simulink model "SYSTEMCOMPLEX"  (R2025b)
settings: Solver=VariableStepAuto  StartTime=0.0  StopTime=10.0  RelTol=1e-3
(part 1 of 2)
settings Model: Creator=GShelton28  LastModifiedBy=GShelton28

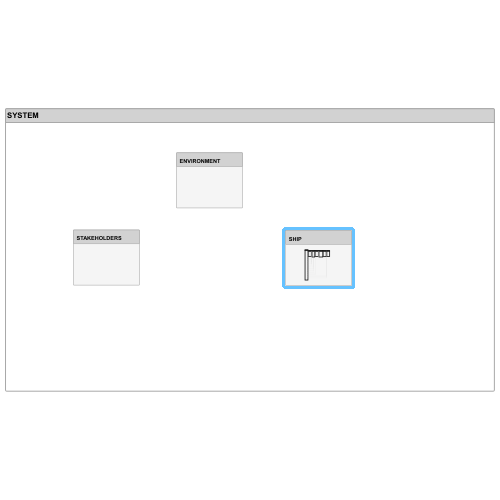
[thumbnail: Simulink's stored preview of the top-level diagram]
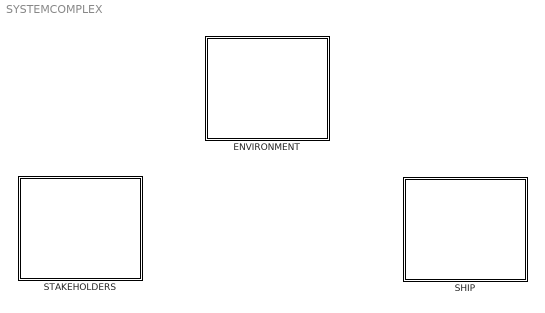
== system SYSTEMCOMPLEX ==
  ENVIRONMENT : Subsystem
      settings: PortSchema="{\"entries\":[{\"content\":{\"headerSize\":26,\"margin\":15,\"minimumSpacing\":25,\"sides\":[{\"content\":{},\"type\":\"ConnectorPlacement.EquallySpacedRectSide\",\"uuid\":\"c62bca68-e99b-4d4a-8c3b-c9a3c6520291\"},{\"content\":{\"side\":\"RIGHT\"},\"type\":\"ConnectorPlacement.EquallySpacedRectSide\",\"uuid\":\"9f78cd75-5645-4950-8d66-9f0d33627f1f\"},{\"content\":{\"side\":\"TOP\"},\"type\":\"ConnectorPlacement.EquallySpacedRectSide\",\"uuid\":\"f95077c9-4a6b-4bf1-8b13-59697d659817\"}]},\"type\":\"ConnectorPlacement.EquallySpacedConnector\",\"uuid\":\"da1ef182-4ed3-4fb4-823f-e8eb0a5ecd15\"}],\"packageUris\":[\"http://schema.mathworks.com/mf0/Connector/R2020b\"],\"version\":\"1.0\"}"
  SHIP : Subsystem
      settings: PortSchema="{\"entries\":[{\"content\":{\"headerSize\":26,\"margin\":15,\"minimumSpacing\":25,\"sides\":[{\"content\":{},\"type\":\"ConnectorPlacement.EquallySpacedRectSide\",\"uuid\":\"c62bca68-e99b-4d4a-8c3b-c9a3c6520291\"},{\"content\":{\"side\":\"RIGHT\"},\"type\":\"ConnectorPlacement.EquallySpacedRectSide\",\"uuid\":\"9f78cd75-5645-4950-8d66-9f0d33627f1f\"},{\"content\":{\"side\":\"TOP\"},\"type\":\"ConnectorPlacement.EquallySpacedRectSide\",\"uuid\":\"f95077c9-4a6b-4bf1-8b13-59697d659817\"}]},\"type\":\"ConnectorPlacement.EquallySpacedConnector\",\"uuid\":\"da1ef182-4ed3-4fb4-823f-e8eb0a5ecd15\"}],\"packageUris\":[\"http://schema.mathworks.com/mf0/Connector/R2020b\"],\"version\":\"1.0\"}"
  STAKEHOLDERS : Subsystem
      settings: PortSchema="{\"entries\":[{\"content\":{\"headerSize\":26,\"margin\":15,\"minimumSpacing\":25,\"sides\":[{\"content\":{},\"type\":\"ConnectorPlacement.EquallySpacedRectSide\",\"uuid\":\"c62bca68-e99b-4d4a-8c3b-c9a3c6520291\"},{\"content\":{\"side\":\"RIGHT\"},\"type\":\"ConnectorPlacement.EquallySpacedRectSide\",\"uuid\":\"9f78cd75-5645-4950-8d66-9f0d33627f1f\"},{\"content\":{\"side\":\"TOP\"},\"type\":\"ConnectorPlacement.EquallySpacedRectSide\",\"uuid\":\"f95077c9-4a6b-4bf1-8b13-59697d659817\"}]},\"type\":\"ConnectorPlacement.EquallySpacedConnector\",\"uuid\":\"da1ef182-4ed3-4fb4-823f-e8eb0a5ecd15\"}],\"packageUris\":[\"http://schema.mathworks.com/mf0/Connector/R2020b\"],\"version\":\"1.0\"}"

== system SYSTEMCOMPLEX/ENVIRONMENT ==

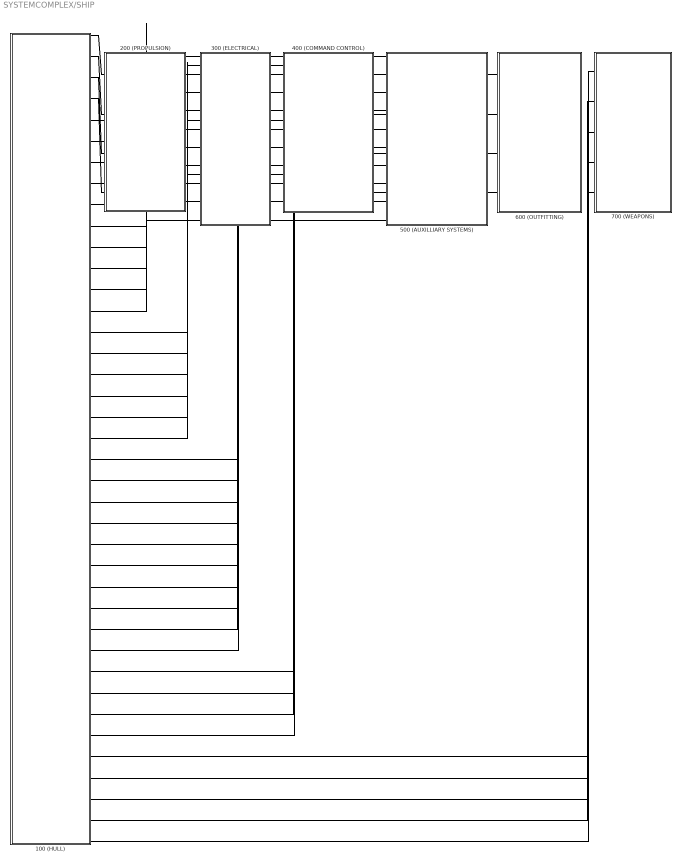
== system SYSTEMCOMPLEX/SHIP ==
  100 (HULL) : Subsystem
      settings: PortSchema="{\"entries\":[{\"content\":{\"headerSize\":26,\"margin\":15,\"minimumSpacing\":25,\"sides\":[{\"content\":{},\"type\":\"ConnectorPlacement.EquallySpacedRectSide\",\"uuid\":\"c62bca68-e99b-4d4a-8c3b-c9a3c6520291\"},{\"content\":{\"connectorIds\":[\"RConn1\",\"RConn2\",\"RConn3\",\"RConn4\",\"RConn5\",\"RConn6\",\"RConn7\",\"RConn8\",\"RConn9\",\"RConn10\",\"RConn11\",\"RConn12\",\"RConn13\",\"RConn14\",\"RConn15\",\"RConn16\",\"RConn17\",\"RConn18\",\"RConn19\",\"RConn20\",\"RConn21\",\"RConn22\",\"RConn23\",\"RConn24\",\"RConn25\",\"RConn26\",\"RConn27\",\"RConn28\",\"RConn29\",\"RConn30\",\"RConn31\",\"RConn32\",\"RConn33\",\"RConn34\",\"RConn35\",\"RConn36\",\"RConn37\",\"RConn38\",\"RConn39\"],\"side\":\"RIGHT\"},\"type\":\"ConnectorPlacement.EquallySpacedRectSide\",\"uuid\":\"9f78cd75-5645-4950-8d66-9f0d33627f1f\"},{\"content\":{\"side\":\"TOP\"},\"type\":\"ConnectorPlacement.EquallySpacedRectSide\",\"uuid\":\"f95077c9-4a6b-4bf1-8b13-59697d659817\"}]},\"type\":\"ConnectorPlacement.EquallySpacedConnector\",\"uuid\":\"da1ef182-4ed3-4fb4-823f-e8eb0a5ecd15\"}],\"packageUris\":[\"http://schema.mathworks.com/mf0/Connector/R2020b\"],\"version\":\"1.0\"}"
  200 (PROPULSION) : Subsystem
      settings: PortSchema="{\"entries\":[{\"content\":{\"headerSize\":26,\"margin\":15,\"minimumSpacing\":25,\"sides\":[{\"content\":{\"connectorIds\":[\"LConn1\",\"LConn2\",\"LConn3\",\"LConn4\"]},\"type\":\"ConnectorPlacement.EquallySpacedRectSide\",\"uuid\":\"c62bca68-e99b-4d4a-8c3b-c9a3c6520291\"},{\"content\":{\"side\":\"RIGHT\"},\"type\":\"ConnectorPlacement.EquallySpacedRectSide\",\"uuid\":\"9f78cd75-5645-4950-8d66-9f0d33627f1f\"},{\"content\":{\"side\":\"TOP\"},\"type\":\"ConnectorPlacement.EquallySpacedRectSide\",\"uuid\":\"f95077c9-4a6b-4bf1-8b13-59697d659817\"}]},\"type\":\"ConnectorPlacement.EquallySpacedConnector\",\"uuid\":\"da1ef182-4ed3-4fb4-823f-e8eb0a5ecd15\"}],\"packageUris\":[\"http://schema.mathworks.com/mf0/Connector/R2020b\"],\"version\":\"1.0\"}"
  300 (ELECTRICAL) : Subsystem
      settings: PortSchema="{\"entries\":[{\"content\":{\"headerSize\":26,\"margin\":15,\"minimumSpacing\":25,\"sides\":[{\"content\":{\"connectorIds\":[\"LConn1\",\"LConn2\",\"LConn3\",\"LConn4\",\"LConn5\",\"LConn6\",\"LConn7\",\"LConn8\",\"LConn9\",\"LConn10\"]},\"type\":\"ConnectorPlacement.EquallySpacedRectSide\",\"uuid\":\"c62bca68-e99b-4d4a-8c3b-c9a3c6520291\"},{\"content\":{\"side\":\"RIGHT\"},\"type\":\"ConnectorPlacement.EquallySpacedRectSide\",\"uuid\":\"9f78cd75-5645-4950-8d66-9f0d33627f1f\"},{\"content\":{\"side\":\"TOP\"},\"type\":\"ConnectorPlacement.EquallySpacedRectSide\",\"uuid\":\"f95077c9-4a6b-4bf1-8b13-59697d659817\"}]},\"type\":\"ConnectorPlacement.EquallySpacedConnector\",\"uuid\":\"da1ef182-4ed3-4fb4-823f-e8eb0a5ecd15\"}],\"packageUris\":[\"http://schema.mathworks.com/mf0/Connector/R2020b\"],\"version\":\"1.0\"}"
  400 (COMMAND CONTROL) : Subsystem
      settings: PortSchema="{\"entries\":[{\"content\":{\"headerSize\":26,\"margin\":15,\"minimumSpacing\":25,\"sides\":[{\"content\":{\"connectorIds\":[\"LConn1\",\"LConn2\",\"LConn3\",\"LConn4\",\"LConn5\",\"LConn6\"]},\"type\":\"ConnectorPlacement.EquallySpacedRectSide\",\"uuid\":\"c62bca68-e99b-4d4a-8c3b-c9a3c6520291\"},{\"content\":{\"side\":\"RIGHT\"},\"type\":\"ConnectorPlacement.EquallySpacedRectSide\",\"uuid\":\"9f78cd75-5645-4950-8d66-9f0d33627f1f\"},{\"content\":{\"side\":\"TOP\"},\"type\":\"ConnectorPlacement.EquallySpacedRectSide\",\"uuid\":\"f95077c9-4a6b-4bf1-8b13-59697d659817\"}]},\"type\":\"ConnectorPlacement.EquallySpacedConnector\",\"uuid\":\"da1ef182-4ed3-4fb4-823f-e8eb0a5ecd15\"}],\"packageUris\":[\"http://schema.mathworks.com/mf0/Connector/R2020b\"],\"version\":\"1.0\"}"
  500 (AUXILLIARY SYSTEMS) : Subsystem
      settings: PortSchema="{\"entries\":[{\"content\":{\"headerSize\":26,\"margin\":15,\"minimumSpacing\":25,\"sides\":[{\"content\":{\"connectorIds\":[\"LConn1\",\"LConn2\",\"LConn3\",\"LConn4\",\"LConn5\",\"LConn6\",\"LConn7\",\"LConn8\",\"LConn9\",\"LConn10\"]},\"type\":\"ConnectorPlacement.EquallySpacedRectSide\",\"uuid\":\"c62bca68-e99b-4d4a-8c3b-c9a3c6520291\"},{\"content\":{\"side\":\"RIGHT\"},\"type\":\"ConnectorPlacement.EquallySpacedRectSide\",\"uuid\":\"9f78cd75-5645-4950-8d66-9f0d33627f1f\"},{\"content\":{\"side\":\"TOP\"},\"type\":\"ConnectorPlacement.EquallySpacedRectSide\",\"uuid\":\"f95077c9-4a6b-4bf1-8b13-59697d659817\"}]},\"type\":\"ConnectorPlacement.EquallySpacedConnector\",\"uuid\":\"da1ef182-4ed3-4fb4-823f-e8eb0a5ecd15\"}],\"packageUris\":[\"http://schema.mathworks.com/mf0/Connector/R2020b\"],\"version\":\"1.0\"}"
  600 (OUTFITTING) : Subsystem
      settings: PortSchema="{\"entries\":[{\"content\":{\"headerSize\":26,\"margin\":15,\"minimumSpacing\":25,\"sides\":[{\"content\":{\"connectorIds\":[\"LConn1\",\"LConn2\",\"LConn3\",\"LConn4\"]},\"type\":\"ConnectorPlacement.EquallySpacedRectSide\",\"uuid\":\"c62bca68-e99b-4d4a-8c3b-c9a3c6520291\"},{\"content\":{\"side\":\"RIGHT\"},\"type\":\"ConnectorPlacement.EquallySpacedRectSide\",\"uuid\":\"9f78cd75-5645-4950-8d66-9f0d33627f1f\"},{\"content\":{\"side\":\"TOP\"},\"type\":\"ConnectorPlacement.EquallySpacedRectSide\",\"uuid\":\"f95077c9-4a6b-4bf1-8b13-59697d659817\"}]},\"type\":\"ConnectorPlacement.EquallySpacedConnector\",\"uuid\":\"da1ef182-4ed3-4fb4-823f-e8eb0a5ecd15\"}],\"packageUris\":[\"http://schema.mathworks.com/mf0/Connector/R2020b\"],\"version\":\"1.0\"}"
  700 (WEAPONS) : Subsystem
      settings: PortSchema="{\"entries\":[{\"content\":{\"headerSize\":26,\"margin\":15,\"minimumSpacing\":25,\"sides\":[{\"content\":{\"connectorIds\":[\"LConn1\",\"LConn2\",\"LConn3\",\"LConn4\",\"LConn5\"]},\"type\":\"ConnectorPlacement.EquallySpacedRectSide\",\"uuid\":\"c62bca68-e99b-4d4a-8c3b-c9a3c6520291\"},{\"content\":{\"side\":\"RIGHT\"},\"type\":\"ConnectorPlacement.EquallySpacedRectSide\",\"uuid\":\"9f78cd75-5645-4950-8d66-9f0d33627f1f\"},{\"content\":{\"side\":\"TOP\"},\"type\":\"ConnectorPlacement.EquallySpacedRectSide\",\"uuid\":\"f95077c9-4a6b-4bf1-8b13-59697d659817\"}]},\"type\":\"ConnectorPlacement.EquallySpacedConnector\",\"uuid\":\"da1ef182-4ed3-4fb4-823f-e8eb0a5ecd15\"}],\"packageUris\":[\"http://schema.mathworks.com/mf0/Connector/R2020b\"],\"version\":\"1.0\"}"
  connections:
  100 (HULL)/RConn1 -- 200 (PROPULSION)/LConn1
  100 (HULL)/RConn2 -- 200 (PROPULSION)/LConn2
  100 (HULL)/RConn3 -- 200 (PROPULSION)/LConn3
  100 (HULL)/RConn4 -- 200 (PROPULSION)/LConn4
  100 (HULL)/RConn5 -- 300 (ELECTRICAL)/LConn1
  100 (HULL)/RConn6 -- 300 (ELECTRICAL)/LConn2
  100 (HULL)/RConn7 -- 300 (ELECTRICAL)/LConn3
  100 (HULL)/RConn8 -- 300 (ELECTRICAL)/LConn4
  100 (HULL)/RConn9 -- 300 (ELECTRICAL)/LConn5
  100 (HULL)/RConn10 -- 300 (ELECTRICAL)/LConn6
  100 (HULL)/RConn11 -- 300 (ELECTRICAL)/LConn7
  100 (HULL)/RConn12 -- 300 (ELECTRICAL)/LConn8
  100 (HULL)/RConn13 -- 300 (ELECTRICAL)/LConn9
  100 (HULL)/RConn14 -- 300 (ELECTRICAL)/LConn10
  100 (HULL)/RConn15 -- 400 (COMMAND CONTROL)/LConn1
  100 (HULL)/RConn16 -- 400 (COMMAND CONTROL)/LConn2
  100 (HULL)/RConn17 -- 400 (COMMAND CONTROL)/LConn3
  100 (HULL)/RConn18 -- 400 (COMMAND CONTROL)/LConn4
  100 (HULL)/RConn19 -- 400 (COMMAND CONTROL)/LConn5
  100 (HULL)/RConn20 -- 400 (COMMAND CONTROL)/LConn6
  500 (AUXILLIARY SYSTEMS)/LConn1 -- 100 (HULL)/RConn21
  100 (HULL)/RConn22 -- 500 (AUXILLIARY SYSTEMS)/LConn2
  100 (HULL)/RConn23 -- 500 (AUXILLIARY SYSTEMS)/LConn3
  100 (HULL)/RConn24 -- 500 (AUXILLIARY SYSTEMS)/LConn4
  500 (AUXILLIARY SYSTEMS)/LConn5 -- 100 (HULL)/RConn25
  100 (HULL)/RConn26 -- 500 (AUXILLIARY SYSTEMS)/LConn6
  500 (AUXILLIARY SYSTEMS)/LConn7 -- 100 (HULL)/RConn27
  100 (HULL)/RConn28 -- 500 (AUXILLIARY SYSTEMS)/LConn8
  500 (AUXILLIARY SYSTEMS)/LConn9 -- 100 (HULL)/RConn29
  100 (HULL)/RConn30 -- 500 (AUXILLIARY SYSTEMS)/LConn10
  600 (OUTFITTING)/LConn1 -- 100 (HULL)/RConn31
  100 (HULL)/RConn32 -- 600 (OUTFITTING)/LConn2
  600 (OUTFITTING)/LConn3 -- 100 (HULL)/RConn33
  100 (HULL)/RConn34 -- 600 (OUTFITTING)/LConn4
  100 (HULL)/RConn35 -- 700 (WEAPONS)/LConn1
  700 (WEAPONS)/LConn2 -- 100 (HULL)/RConn36
  100 (HULL)/RConn37 -- 700 (WEAPONS)/LConn3
  700 (WEAPONS)/LConn4 -- 100 (HULL)/RConn38
  100 (HULL)/RConn39 -- 700 (WEAPONS)/LConn5

== system SYSTEMCOMPLEX/STAKEHOLDERS ==

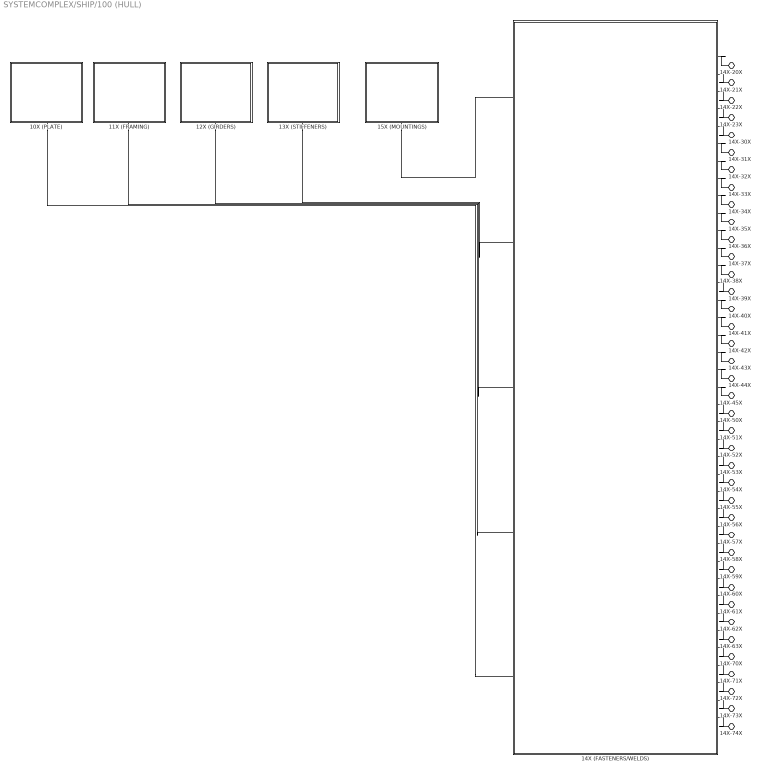
== system SYSTEMCOMPLEX/SHIP/100 (HULL) ==
  10X (PLATE) : Subsystem
      settings: PortSchema="{\"entries\":[{\"content\":{\"headerSize\":26,\"margin\":15,\"minimumSpacing\":25,\"sides\":[{\"content\":{},\"type\":\"ConnectorPlacement.EquallySpacedRectSide\",\"uuid\":\"c62bca68-e99b-4d4a-8c3b-c9a3c6520291\"},{\"content\":{\"side\":\"RIGHT\"},\"type\":\"ConnectorPlacement.EquallySpacedRectSide\",\"uuid\":\"9f78cd75-5645-4950-8d66-9f0d33627f1f\"},{\"content\":{\"side\":\"TOP\"},\"type\":\"ConnectorPlacement.EquallySpacedRectSide\",\"uuid\":\"f95077c9-4a6b-4bf1-8b13-59697d659817\"},{\"content\":{\"connectorIds\":[\"RConn1\"],\"side\":\"BOTTOM\"},\"type\":\"ConnectorPlacement.EquallySpacedRectSide\",\"uuid\":\"ddd19866-59cb-4aa8-acfa-d5f465b87cbd\"}]},\"type\":\"ConnectorPlacement.EquallySpacedConnector\",\"uuid\":\"da1ef182-4ed3-4fb4-823f-e8eb0a5ecd15\"}],\"packageUris\":[\"http://schema.mathworks.com/mf0/Connector/R2020b\"],\"version\":\"1.0\"}"
  11X (FRAMING) : Subsystem
      settings: PortSchema="{\"entries\":[{\"content\":{\"headerSize\":26,\"margin\":15,\"minimumSpacing\":25,\"sides\":[{\"content\":{},\"type\":\"ConnectorPlacement.EquallySpacedRectSide\",\"uuid\":\"c62bca68-e99b-4d4a-8c3b-c9a3c6520291\"},{\"content\":{\"side\":\"RIGHT\"},\"type\":\"ConnectorPlacement.EquallySpacedRectSide\",\"uuid\":\"9f78cd75-5645-4950-8d66-9f0d33627f1f\"},{\"content\":{\"side\":\"TOP\"},\"type\":\"ConnectorPlacement.EquallySpacedRectSide\",\"uuid\":\"f95077c9-4a6b-4bf1-8b13-59697d659817\"},{\"content\":{\"connectorIds\":[\"RConn1\"],\"side\":\"BOTTOM\"},\"type\":\"ConnectorPlacement.EquallySpacedRectSide\",\"uuid\":\"e30eef64-4d31-47ea-aab5-fe3e5ba0a546\"}]},\"type\":\"ConnectorPlacement.EquallySpacedConnector\",\"uuid\":\"da1ef182-4ed3-4fb4-823f-e8eb0a5ecd15\"}],\"packageUris\":[\"http://schema.mathworks.com/mf0/Connector/R2020b\"],\"version\":\"1.0\"}"
  12X (GIRDERS) : Subsystem
      settings: PortSchema="{\"entries\":[{\"content\":{\"headerSize\":26,\"margin\":15,\"minimumSpacing\":25,\"sides\":[{\"content\":{},\"type\":\"ConnectorPlacement.EquallySpacedRectSide\",\"uuid\":\"c62bca68-e99b-4d4a-8c3b-c9a3c6520291\"},{\"content\":{\"side\":\"RIGHT\"},\"type\":\"ConnectorPlacement.EquallySpacedRectSide\",\"uuid\":\"9f78cd75-5645-4950-8d66-9f0d33627f1f\"},{\"content\":{\"side\":\"TOP\"},\"type\":\"ConnectorPlacement.EquallySpacedRectSide\",\"uuid\":\"f95077c9-4a6b-4bf1-8b13-59697d659817\"},{\"content\":{\"connectorIds\":[\"RConn1\"],\"side\":\"BOTTOM\"},\"type\":\"ConnectorPlacement.EquallySpacedRectSide\",\"uuid\":\"1e29fe40-13d2-4b8b-aa86-0c115e4d1338\"}]},\"type\":\"ConnectorPlacement.EquallySpacedConnector\",\"uuid\":\"da1ef182-4ed3-4fb4-823f-e8eb0a5ecd15\"}],\"packageUris\":[\"http://schema.mathworks.com/mf0/Connector/R2020b\"],\"version\":\"1.0\"}"
  13X (STIFFENERS) : Subsystem
      settings: PortSchema="{\"entries\":[{\"content\":{\"headerSize\":26,\"margin\":15,\"minimumSpacing\":25,\"sides\":[{\"content\":{},\"type\":\"ConnectorPlacement.EquallySpacedRectSide\",\"uuid\":\"c62bca68-e99b-4d4a-8c3b-c9a3c6520291\"},{\"content\":{\"side\":\"RIGHT\"},\"type\":\"ConnectorPlacement.EquallySpacedRectSide\",\"uuid\":\"9f78cd75-5645-4950-8d66-9f0d33627f1f\"},{\"content\":{\"side\":\"TOP\"},\"type\":\"ConnectorPlacement.EquallySpacedRectSide\",\"uuid\":\"f95077c9-4a6b-4bf1-8b13-59697d659817\"},{\"content\":{\"connectorIds\":[\"RConn1\"],\"side\":\"BOTTOM\"},\"type\":\"ConnectorPlacement.EquallySpacedRectSide\",\"uuid\":\"7faf6a59-0ecd-4c67-a0ee-65a3195c0019\"}]},\"type\":\"ConnectorPlacement.EquallySpacedConnector\",\"uuid\":\"da1ef182-4ed3-4fb4-823f-e8eb0a5ecd15\"}],\"packageUris\":[\"http://schema.mathworks.com/mf0/Connector/R2020b\"],\"version\":\"1.0\"}"
  14X (FASTENERS/WELDS) : Subsystem
      settings: PortSchema="{\"entries\":[{\"content\":{\"headerSize\":26,\"margin\":15,\"minimumSpacing\":25,\"sides\":[{\"content\":{\"connectorIds\":[\"LConn1\",\"LConn2\",\"LConn3\",\"LConn4\",\"LConn5\"]},\"type\":\"ConnectorPlacement.EquallySpacedRectSide\",\"uuid\":\"c62bca68-e99b-4d4a-8c3b-c9a3c6520291\"},{\"content\":{\"connectorIds\":[\"RConn1\",\"RConn2\",\"RConn3\",\"RConn4\",\"RConn5\",\"RConn6\",\"RConn7\",\"RConn8\",\"RConn9\",\"RConn10\",\"RConn11\",\"RConn12\",\"RConn13\",\"RConn14\",\"RConn15\",\"RConn16\",\"RConn17\",\"RConn18\",\"RConn19\",\"RConn20\",\"RConn21\",\"RConn22\",\"RConn23\",\"RConn24\",\"RConn25\",\"RConn26\",\"RConn27\",\"RConn28\",\"RConn29\",\"RConn30\",\"RConn31\",\"RConn32\",\"RConn33\",\"RConn34\",\"RConn35\",\"RConn36\",\"RConn37\",\"RConn38\",\"RConn39\"],\"side\":\"RIGHT\"},\"type\":\"ConnectorPlacement.EquallySpacedRectSide\",\"uuid\":\"9f78cd75-5645-4950-8d66-9f0d33627f1f\"},{\"content\":{\"side\":\"TOP\"},\"type\":\"ConnectorPlacement.EquallySpacedRectSide\",\"uuid\":\"f95077c9-4a6b-4bf1-8b13-59697d659817\"},{\"content\":{\"side\":\"BOTTOM\"},\"type\":\"ConnectorPlacement.EquallySpacedRectSide\",\"uuid\":\"eacd5ff9-c8c4-4550-88da-b1bfe7e72945\"}]},\"type\":\"ConnectorPlacement.EquallySpacedConnector\",\"uuid\":\"da1ef182-4ed3-4fb4-823f-e8eb0a5ecd15\"}],\"packageUris\":[\"http://schema.mathworks.com/mf0/Connector/R2020b\"],\"version\":\"1.0\"}"
  15X (MOUNTINGS) : Subsystem
      settings: PortSchema="{\"entries\":[{\"content\":{\"headerSize\":26,\"margin\":15,\"minimumSpacing\":25,\"sides\":[{\"content\":{},\"type\":\"ConnectorPlacement.EquallySpacedRectSide\",\"uuid\":\"c62bca68-e99b-4d4a-8c3b-c9a3c6520291\"},{\"content\":{\"side\":\"RIGHT\"},\"type\":\"ConnectorPlacement.EquallySpacedRectSide\",\"uuid\":\"9f78cd75-5645-4950-8d66-9f0d33627f1f\"},{\"content\":{\"side\":\"TOP\"},\"type\":\"ConnectorPlacement.EquallySpacedRectSide\",\"uuid\":\"f95077c9-4a6b-4bf1-8b13-59697d659817\"},{\"content\":{\"connectorIds\":[\"RConn1\"],\"side\":\"BOTTOM\"},\"type\":\"ConnectorPlacement.EquallySpacedRectSide\",\"uuid\":\"0aa2e608-037e-43d9-a7e9-e80277dde91c\"}]},\"type\":\"ConnectorPlacement.EquallySpacedConnector\",\"uuid\":\"da1ef182-4ed3-4fb4-823f-e8eb0a5ecd15\"}],\"packageUris\":[\"http://schema.mathworks.com/mf0/Connector/R2020b\"],\"version\":\"1.0\"}"
  14X-20X : PMIOPort  Side=Right
  14X-21X : PMIOPort  Port=2  Side=Right
  14X-22X : PMIOPort  Port=3  Side=Right
  14X-23X : PMIOPort  Port=4  Side=Right
  14X-30X : PMIOPort  Port=5  Side=Right
  14X-31X : PMIOPort  Port=6  Side=Right
  14X-32X : PMIOPort  Port=7  Side=Right
  14X-33X : PMIOPort  Port=8  Side=Right
  14X-34X : PMIOPort  Port=9  Side=Right
  14X-35X : PMIOPort  Port=10  Side=Right
  14X-36X : PMIOPort  Port=11  Side=Right
  14X-37X : PMIOPort  Port=12  Side=Right
  14X-38X : PMIOPort  Port=13  Side=Right
  14X-39X : PMIOPort  Port=14  Side=Right
  14X-40X : PMIOPort  Port=15  Side=Right
  14X-41X : PMIOPort  Port=16  Side=Right
  14X-42X : PMIOPort  Port=17  Side=Right
  14X-43X : PMIOPort  Port=18  Side=Right
  14X-44X : PMIOPort  Port=19  Side=Right
  14X-45X : PMIOPort  Port=20  Side=Right
  14X-50X : PMIOPort  Port=21  Side=Right
  14X-51X : PMIOPort  Port=22  Side=Right
  14X-52X : PMIOPort  Port=23  Side=Right
  14X-53X : PMIOPort  Port=24  Side=Right
  14X-54X : PMIOPort  Port=25  Side=Right
  14X-55X : PMIOPort  Port=26  Side=Right
  14X-56X : PMIOPort  Port=27  Side=Right
  14X-57X : PMIOPort  Port=28  Side=Right
  14X-58X : PMIOPort  Port=29  Side=Right
  14X-59X : PMIOPort  Port=30  Side=Right
  14X-60X : PMIOPort  Port=31  Side=Right
  14X-61X : PMIOPort  Port=32  Side=Right
  14X-62X : PMIOPort  Port=33  Side=Right
  14X-63X : PMIOPort  Port=34  Side=Right
  14X-70X : PMIOPort  Port=35  Side=Right
  14X-71X : PMIOPort  Port=36  Side=Right
  14X-72X : PMIOPort  Port=37  Side=Right
  14X-73X : PMIOPort  Port=38  Side=Right
  14X-74X : PMIOPort  Port=39  Side=Right
  connections:
  10X (PLATE)/RConn1 -- 14X (FASTENERS/WELDS)/LConn5
  11X (FRAMING)/RConn1 -- 14X (FASTENERS/WELDS)/LConn4
  12X (GIRDERS)/RConn1 -- 14X (FASTENERS/WELDS)/LConn3
  13X (STIFFENERS)/RConn1 -- 14X (FASTENERS/WELDS)/LConn2
  15X (MOUNTINGS)/RConn1 -- 14X (FASTENERS/WELDS)/LConn1
  14X (FASTENERS/WELDS)/RConn1 -- 14X-20X/RConn1
  14X-21X/RConn1 -- 14X (FASTENERS/WELDS)/RConn2
  14X-22X/RConn1 -- 14X (FASTENERS/WELDS)/RConn3
  14X-23X/RConn1 -- 14X (FASTENERS/WELDS)/RConn4
  14X-30X/RConn1 -- 14X (FASTENERS/WELDS)/RConn5
  14X (FASTENERS/WELDS)/RConn6 -- 14X-31X/RConn1
  14X (FASTENERS/WELDS)/RConn7 -- 14X-32X/RConn1
  14X (FASTENERS/WELDS)/RConn8 -- 14X-33X/RConn1
  14X (FASTENERS/WELDS)/RConn9 -- 14X-34X/RConn1
  14X (FASTENERS/WELDS)/RConn10 -- 14X-35X/RConn1
  14X (FASTENERS/WELDS)/RConn11 -- 14X-36X/RConn1
  14X (FASTENERS/WELDS)/RConn12 -- 14X-37X/RConn1
  14X (FASTENERS/WELDS)/RConn13 -- 14X-38X/RConn1
  14X (FASTENERS/WELDS)/RConn15 -- 14X-40X/RConn1
  14X (FASTENERS/WELDS)/RConn16 -- 14X-41X/RConn1
  14X (FASTENERS/WELDS)/RConn17 -- 14X-42X/RConn1
  14X (FASTENERS/WELDS)/RConn18 -- 14X-43X/RConn1
  14X (FASTENERS/WELDS)/RConn19 -- 14X-44X/RConn1
  14X (FASTENERS/WELDS)/RConn20 -- 14X-45X/RConn1
  14X-50X/RConn1 -- 14X (FASTENERS/WELDS)/RConn21
  14X-51X/RConn1 -- 14X (FASTENERS/WELDS)/RConn22
  14X-52X/RConn1 -- 14X (FASTENERS/WELDS)/RConn23
  14X-53X/RConn1 -- 14X (FASTENERS/WELDS)/RConn24
  14X-54X/RConn1 -- 14X (FASTENERS/WELDS)/RConn25
  14X-55X/RConn1 -- 14X (FASTENERS/WELDS)/RConn26
  14X-56X/RConn1 -- 14X (FASTENERS/WELDS)/RConn27
  14X-57X/RConn1 -- 14X (FASTENERS/WELDS)/RConn28
  14X-58X/RConn1 -- 14X (FASTENERS/WELDS)/RConn29
  14X-59X/RConn1 -- 14X (FASTENERS/WELDS)/RConn30
  14X-60X/RConn1 -- 14X (FASTENERS/WELDS)/RConn31
  14X-61X/RConn1 -- 14X (FASTENERS/WELDS)/RConn32
  14X-62X/RConn1 -- 14X (FASTENERS/WELDS)/RConn33
  14X-63X/RConn1 -- 14X (FASTENERS/WELDS)/RConn34
  14X-70X/RConn1 -- 14X (FASTENERS/WELDS)/RConn35
  14X-71X/RConn1 -- 14X (FASTENERS/WELDS)/RConn36
  14X-72X/RConn1 -- 14X (FASTENERS/WELDS)/RConn37
  14X-73X/RConn1 -- 14X (FASTENERS/WELDS)/RConn38
  14X-74X/RConn1 -- 14X (FASTENERS/WELDS)/RConn39
  14X-39X/RConn1 -- 14X (FASTENERS/WELDS)/RConn14

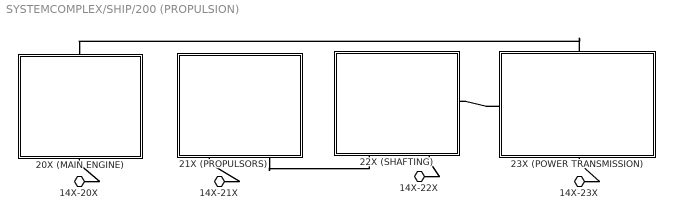
== system SYSTEMCOMPLEX/SHIP/200 (PROPULSION) ==
  20X (MAIN ENGINE) : Subsystem
      settings: PortSchema="{\"entries\":[{\"content\":{\"headerSize\":26,\"margin\":15,\"minimumSpacing\":25,\"sides\":[{\"content\":{},\"type\":\"ConnectorPlacement.EquallySpacedRectSide\",\"uuid\":\"c62bca68-e99b-4d4a-8c3b-c9a3c6520291\"},{\"content\":{\"side\":\"RIGHT\"},\"type\":\"ConnectorPlacement.EquallySpacedRectSide\",\"uuid\":\"9f78cd75-5645-4950-8d66-9f0d33627f1f\"},{\"content\":{\"connectorIds\":[\"LConn2\"],\"side\":\"TOP\"},\"type\":\"ConnectorPlacement.EquallySpacedRectSide\",\"uuid\":\"f95077c9-4a6b-4bf1-8b13-59697d659817\"},{\"content\":{\"connectorIds\":[\"LConn1\"],\"side\":\"BOTTOM\"},\"type\":\"ConnectorPlacement.EquallySpacedRectSide\",\"uuid\":\"1ff1dd93-edda-475a-b328-5828db0b6df2\"}]},\"type\":\"ConnectorPlacement.EquallySpacedConnector\",\"uuid\":\"da1ef182-4ed3-4fb4-823f-e8eb0a5ecd15\"}],\"packageUris\":[\"http://schema.mathworks.com/mf0/Connector/R2020b\"],\"version\":\"1.0\"}"
  21X (PROPULSORS) : Subsystem
      settings: PortSchema="{\"entries\":[{\"content\":{\"headerSize\":26,\"margin\":15,\"minimumSpacing\":25,\"sides\":[{\"content\":{},\"type\":\"ConnectorPlacement.EquallySpacedRectSide\",\"uuid\":\"c62bca68-e99b-4d4a-8c3b-c9a3c6520291\"},{\"content\":{\"side\":\"RIGHT\"},\"type\":\"ConnectorPlacement.EquallySpacedRectSide\",\"uuid\":\"9f78cd75-5645-4950-8d66-9f0d33627f1f\"},{\"content\":{\"side\":\"TOP\"},\"type\":\"ConnectorPlacement.EquallySpacedRectSide\",\"uuid\":\"f95077c9-4a6b-4bf1-8b13-59697d659817\"},{\"content\":{\"connectorIds\":[\"RConn1\",\"RConn2\"],\"side\":\"BOTTOM\"},\"type\":\"ConnectorPlacement.EquallySpacedRectSide\",\"uuid\":\"6b5f2b68-9ed2-4485-9686-f8a23585a666\"}]},\"type\":\"ConnectorPlacement.EquallySpacedConnector\",\"uuid\":\"da1ef182-4ed3-4fb4-823f-e8eb0a5ecd15\"}],\"packageUris\":[\"http://schema.mathworks.com/mf0/Connector/R2020b\"],\"version\":\"1.0\"}"
  22X (SHAFTING) : Subsystem
      settings: PortSchema="{\"entries\":[{\"content\":{\"headerSize\":26,\"margin\":15,\"minimumSpacing\":25,\"sides\":[{\"content\":{},\"type\":\"ConnectorPlacement.EquallySpacedRectSide\",\"uuid\":\"c62bca68-e99b-4d4a-8c3b-c9a3c6520291\"},{\"content\":{\"connectorIds\":[\"RConn1\"],\"side\":\"RIGHT\"},\"type\":\"ConnectorPlacement.EquallySpacedRectSide\",\"uuid\":\"9f78cd75-5645-4950-8d66-9f0d33627f1f\"},{\"content\":{\"side\":\"TOP\"},\"type\":\"ConnectorPlacement.EquallySpacedRectSide\",\"uuid\":\"f95077c9-4a6b-4bf1-8b13-59697d659817\"},{\"content\":{\"connectorIds\":[\"RConn3\",\"RConn2\"],\"side\":\"BOTTOM\"},\"type\":\"ConnectorPlacement.EquallySpacedRectSide\",\"uuid\":\"1f93f758-4269-498d-aa3c-a1654d57bbcc\"}]},\"type\":\"ConnectorPlacement.EquallySpacedConnector\",\"uuid\":\"da1ef182-4ed3-4fb4-823f-e8eb0a5ecd15\"}],\"packageUris\":[\"http://schema.mathworks.com/mf0/Connector/R2020b\"],\"version\":\"1.0\"}"
  23X (POWER TRANSMISSION) : Subsystem
      settings: PortSchema="{\"entries\":[{\"content\":{\"headerSize\":26,\"margin\":15,\"minimumSpacing\":25,\"sides\":[{\"content\":{\"connectorIds\":[\"LConn1\"]},\"type\":\"ConnectorPlacement.EquallySpacedRectSide\",\"uuid\":\"c62bca68-e99b-4d4a-8c3b-c9a3c6520291\"},{\"content\":{\"side\":\"RIGHT\"},\"type\":\"ConnectorPlacement.EquallySpacedRectSide\",\"uuid\":\"9f78cd75-5645-4950-8d66-9f0d33627f1f\"},{\"content\":{\"connectorIds\":[\"LConn2\"],\"side\":\"TOP\"},\"type\":\"ConnectorPlacement.EquallySpacedRectSide\",\"uuid\":\"f95077c9-4a6b-4bf1-8b13-59697d659817\"},{\"content\":{\"connectorIds\":[\"RConn1\"],\"side\":\"BOTTOM\"},\"type\":\"ConnectorPlacement.EquallySpacedRectSide\",\"uuid\":\"886e986c-d088-4ccd-a11a-30cba32770e8\"}]},\"type\":\"ConnectorPlacement.EquallySpacedConnector\",\"uuid\":\"da1ef182-4ed3-4fb4-823f-e8eb0a5ecd15\"}],\"packageUris\":[\"http://schema.mathworks.com/mf0/Connector/R2020b\"],\"version\":\"1.0\"}"
  14X-20X : PMIOPort  Side=Left
  14X-21X : PMIOPort  Port=2  Side=Left
  14X-22X : PMIOPort  Port=3  Side=Left
  14X-23X : PMIOPort  Port=4  Side=Left
  connections:
  23X (POWER TRANSMISSION)/LConn2 -- 20X (MAIN ENGINE)/LConn2
  21X (PROPULSORS)/RConn2 -- 22X (SHAFTING)/RConn3
  23X (POWER TRANSMISSION)/LConn1 -- 22X (SHAFTING)/RConn1
  14X-20X/RConn1 -- 20X (MAIN ENGINE)/LConn1
  14X-21X/RConn1 -- 21X (PROPULSORS)/RConn1
  14X-22X/RConn1 -- 22X (SHAFTING)/RConn2
  14X-23X/RConn1 -- 23X (POWER TRANSMISSION)/RConn1

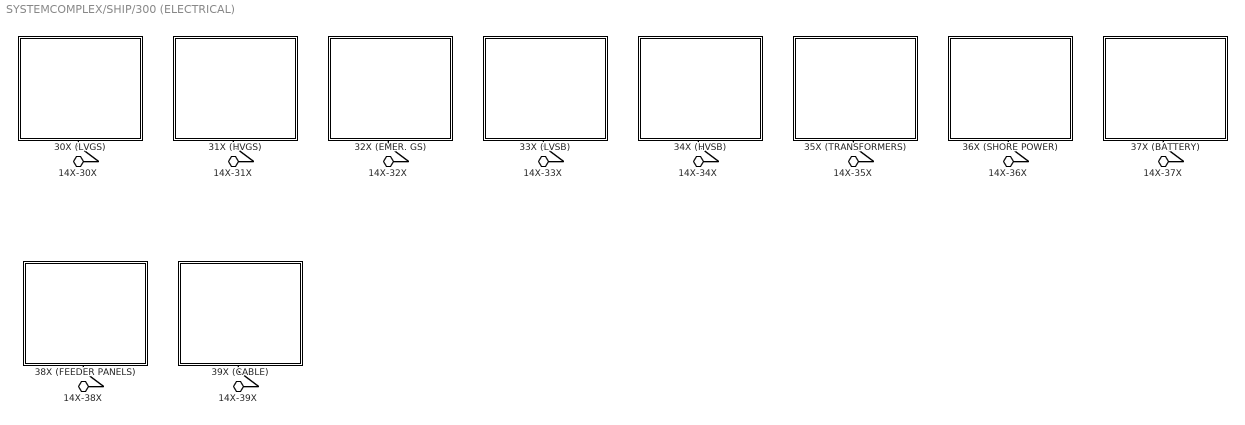
== system SYSTEMCOMPLEX/SHIP/300 (ELECTRICAL) ==
  30X (LVGS) : Subsystem
      settings: PortSchema="{\"entries\":[{\"content\":{\"headerSize\":26,\"margin\":15,\"minimumSpacing\":25,\"sides\":[{\"content\":{},\"type\":\"ConnectorPlacement.EquallySpacedRectSide\",\"uuid\":\"c62bca68-e99b-4d4a-8c3b-c9a3c6520291\"},{\"content\":{\"side\":\"RIGHT\"},\"type\":\"ConnectorPlacement.EquallySpacedRectSide\",\"uuid\":\"9f78cd75-5645-4950-8d66-9f0d33627f1f\"},{\"content\":{\"side\":\"TOP\"},\"type\":\"ConnectorPlacement.EquallySpacedRectSide\",\"uuid\":\"f95077c9-4a6b-4bf1-8b13-59697d659817\"},{\"content\":{\"connectorIds\":[\"RConn1\"],\"side\":\"BOTTOM\"},\"type\":\"ConnectorPlacement.EquallySpacedRectSide\",\"uuid\":\"264ceb2d-2194-473f-bd49-42333d529a66\"}]},\"type\":\"ConnectorPlacement.EquallySpacedConnector\",\"uuid\":\"da1ef182-4ed3-4fb4-823f-e8eb0a5ecd15\"}],\"packageUris\":[\"http://schema.mathworks.com/mf0/Connector/R2020b\"],\"version\":\"1.0\"}"
  31X (HVGS) : Subsystem
      settings: PortSchema="{\"entries\":[{\"content\":{\"headerSize\":26,\"margin\":15,\"minimumSpacing\":25,\"sides\":[{\"content\":{},\"type\":\"ConnectorPlacement.EquallySpacedRectSide\",\"uuid\":\"c62bca68-e99b-4d4a-8c3b-c9a3c6520291\"},{\"content\":{\"side\":\"RIGHT\"},\"type\":\"ConnectorPlacement.EquallySpacedRectSide\",\"uuid\":\"9f78cd75-5645-4950-8d66-9f0d33627f1f\"},{\"content\":{\"side\":\"TOP\"},\"type\":\"ConnectorPlacement.EquallySpacedRectSide\",\"uuid\":\"f95077c9-4a6b-4bf1-8b13-59697d659817\"},{\"content\":{\"connectorIds\":[\"RConn1\"],\"side\":\"BOTTOM\"},\"type\":\"ConnectorPlacement.EquallySpacedRectSide\",\"uuid\":\"f6dd318a-df87-4470-894a-05aa0d1c9a62\"}]},\"type\":\"ConnectorPlacement.EquallySpacedConnector\",\"uuid\":\"da1ef182-4ed3-4fb4-823f-e8eb0a5ecd15\"}],\"packageUris\":[\"http://schema.mathworks.com/mf0/Connector/R2020b\"],\"version\":\"1.0\"}"
  32X (EMER. GS) : Subsystem
      settings: PortSchema="{\"entries\":[{\"content\":{\"headerSize\":26,\"margin\":15,\"minimumSpacing\":25,\"sides\":[{\"content\":{},\"type\":\"ConnectorPlacement.EquallySpacedRectSide\",\"uuid\":\"c62bca68-e99b-4d4a-8c3b-c9a3c6520291\"},{\"content\":{\"side\":\"RIGHT\"},\"type\":\"ConnectorPlacement.EquallySpacedRectSide\",\"uuid\":\"9f78cd75-5645-4950-8d66-9f0d33627f1f\"},{\"content\":{\"side\":\"TOP\"},\"type\":\"ConnectorPlacement.EquallySpacedRectSide\",\"uuid\":\"f95077c9-4a6b-4bf1-8b13-59697d659817\"},{\"content\":{\"connectorIds\":[\"RConn1\"],\"side\":\"BOTTOM\"},\"type\":\"ConnectorPlacement.EquallySpacedRectSide\",\"uuid\":\"3a1d08c9-370f-4ab6-aa25-1f67b2c1fd59\"}]},\"type\":\"ConnectorPlacement.EquallySpacedConnector\",\"uuid\":\"da1ef182-4ed3-4fb4-823f-e8eb0a5ecd15\"}],\"packageUris\":[\"http://schema.mathworks.com/mf0/Connector/R2020b\"],\"version\":\"1.0\"}"
  33X (LVSB) : Subsystem
      settings: PortSchema="{\"entries\":[{\"content\":{\"headerSize\":26,\"margin\":15,\"minimumSpacing\":25,\"sides\":[{\"content\":{},\"type\":\"ConnectorPlacement.EquallySpacedRectSide\",\"uuid\":\"c62bca68-e99b-4d4a-8c3b-c9a3c6520291\"},{\"content\":{\"side\":\"RIGHT\"},\"type\":\"ConnectorPlacement.EquallySpacedRectSide\",\"uuid\":\"9f78cd75-5645-4950-8d66-9f0d33627f1f\"},{\"content\":{\"side\":\"TOP\"},\"type\":\"ConnectorPlacement.EquallySpacedRectSide\",\"uuid\":\"f95077c9-4a6b-4bf1-8b13-59697d659817\"},{\"content\":{\"connectorIds\":[\"RConn1\"],\"side\":\"BOTTOM\"},\"type\":\"ConnectorPlacement.EquallySpacedRectSide\",\"uuid\":\"7c8141e3-2141-4bb3-89bd-e025a2a4dcbf\"}]},\"type\":\"ConnectorPlacement.EquallySpacedConnector\",\"uuid\":\"da1ef182-4ed3-4fb4-823f-e8eb0a5ecd15\"}],\"packageUris\":[\"http://schema.mathworks.com/mf0/Connector/R2020b\"],\"version\":\"1.0\"}"
  34X (HVSB) : Subsystem
      settings: PortSchema="{\"entries\":[{\"content\":{\"headerSize\":26,\"margin\":15,\"minimumSpacing\":25,\"sides\":[{\"content\":{},\"type\":\"ConnectorPlacement.EquallySpacedRectSide\",\"uuid\":\"c62bca68-e99b-4d4a-8c3b-c9a3c6520291\"},{\"content\":{\"side\":\"RIGHT\"},\"type\":\"ConnectorPlacement.EquallySpacedRectSide\",\"uuid\":\"9f78cd75-5645-4950-8d66-9f0d33627f1f\"},{\"content\":{\"side\":\"TOP\"},\"type\":\"ConnectorPlacement.EquallySpacedRectSide\",\"uuid\":\"f95077c9-4a6b-4bf1-8b13-59697d659817\"},{\"content\":{\"connectorIds\":[\"RConn1\"],\"side\":\"BOTTOM\"},\"type\":\"ConnectorPlacement.EquallySpacedRectSide\",\"uuid\":\"cfdef2ea-cf08-493a-8830-0ab88c080493\"}]},\"type\":\"ConnectorPlacement.EquallySpacedConnector\",\"uuid\":\"da1ef182-4ed3-4fb4-823f-e8eb0a5ecd15\"}],\"packageUris\":[\"http://schema.mathworks.com/mf0/Connector/R2020b\"],\"version\":\"1.0\"}"
  35X (TRANSFORMERS) : Subsystem
      settings: PortSchema="{\"entries\":[{\"content\":{\"headerSize\":26,\"margin\":15,\"minimumSpacing\":25,\"sides\":[{\"content\":{},\"type\":\"ConnectorPlacement.EquallySpacedRectSide\",\"uuid\":\"c62bca68-e99b-4d4a-8c3b-c9a3c6520291\"},{\"content\":{\"side\":\"RIGHT\"},\"type\":\"ConnectorPlacement.EquallySpacedRectSide\",\"uuid\":\"9f78cd75-5645-4950-8d66-9f0d33627f1f\"},{\"content\":{\"side\":\"TOP\"},\"type\":\"ConnectorPlacement.EquallySpacedRectSide\",\"uuid\":\"f95077c9-4a6b-4bf1-8b13-59697d659817\"},{\"content\":{\"connectorIds\":[\"RConn1\"],\"side\":\"BOTTOM\"},\"type\":\"ConnectorPlacement.EquallySpacedRectSide\",\"uuid\":\"a7a87ab0-1a77-44d6-9921-825152163c35\"}]},\"type\":\"ConnectorPlacement.EquallySpacedConnector\",\"uuid\":\"da1ef182-4ed3-4fb4-823f-e8eb0a5ecd15\"}],\"packageUris\":[\"http://schema.mathworks.com/mf0/Connector/R2020b\"],\"version\":\"1.0\"}"
  36X (SHORE POWER) : Subsystem
      settings: PortSchema="{\"entries\":[{\"content\":{\"headerSize\":26,\"margin\":15,\"minimumSpacing\":25,\"sides\":[{\"content\":{},\"type\":\"ConnectorPlacement.EquallySpacedRectSide\",\"uuid\":\"c62bca68-e99b-4d4a-8c3b-c9a3c6520291\"},{\"content\":{\"side\":\"RIGHT\"},\"type\":\"ConnectorPlacement.EquallySpacedRectSide\",\"uuid\":\"9f78cd75-5645-4950-8d66-9f0d33627f1f\"},{\"content\":{\"side\":\"TOP\"},\"type\":\"ConnectorPlacement.EquallySpacedRectSide\",\"uuid\":\"f95077c9-4a6b-4bf1-8b13-59697d659817\"},{\"content\":{\"connectorIds\":[\"RConn1\"],\"side\":\"BOTTOM\"},\"type\":\"ConnectorPlacement.EquallySpacedRectSide\",\"uuid\":\"98d15bf2-7595-4bb3-8038-5dc9c6428161\"}]},\"type\":\"ConnectorPlacement.EquallySpacedConnector\",\"uuid\":\"da1ef182-4ed3-4fb4-823f-e8eb0a5ecd15\"}],\"packageUris\":[\"http://schema.mathworks.com/mf0/Connector/R2020b\"],\"version\":\"1.0\"}"
  37X (BATTERY) : Subsystem
      settings: PortSchema="{\"entries\":[{\"content\":{\"headerSize\":26,\"margin\":15,\"minimumSpacing\":25,\"sides\":[{\"content\":{},\"type\":\"ConnectorPlacement.EquallySpacedRectSide\",\"uuid\":\"c62bca68-e99b-4d4a-8c3b-c9a3c6520291\"},{\"content\":{\"side\":\"RIGHT\"},\"type\":\"ConnectorPlacement.EquallySpacedRectSide\",\"uuid\":\"9f78cd75-5645-4950-8d66-9f0d33627f1f\"},{\"content\":{\"side\":\"TOP\"},\"type\":\"ConnectorPlacement.EquallySpacedRectSide\",\"uuid\":\"f95077c9-4a6b-4bf1-8b13-59697d659817\"},{\"content\":{\"connectorIds\":[\"RConn1\"],\"side\":\"BOTTOM\"},\"type\":\"ConnectorPlacement.EquallySpacedRectSide\",\"uuid\":\"28cd9019-8f63-4d9a-829c-4dc13ebdc12a\"}]},\"type\":\"ConnectorPlacement.EquallySpacedConnector\",\"uuid\":\"da1ef182-4ed3-4fb4-823f-e8eb0a5ecd15\"}],\"packageUris\":[\"http://schema.mathworks.com/mf0/Connector/R2020b\"],\"version\":\"1.0\"}"
  38X (FEEDER PANELS) : Subsystem
      settings: PortSchema="{\"entries\":[{\"content\":{\"headerSize\":26,\"margin\":15,\"minimumSpacing\":25,\"sides\":[{\"content\":{},\"type\":\"ConnectorPlacement.EquallySpacedRectSide\",\"uuid\":\"c62bca68-e99b-4d4a-8c3b-c9a3c6520291\"},{\"content\":{\"side\":\"RIGHT\"},\"type\":\"ConnectorPlacement.EquallySpacedRectSide\",\"uuid\":\"9f78cd75-5645-4950-8d66-9f0d33627f1f\"},{\"content\":{\"side\":\"TOP\"},\"type\":\"ConnectorPlacement.EquallySpacedRectSide\",\"uuid\":\"f95077c9-4a6b-4bf1-8b13-59697d659817\"},{\"content\":{\"connectorIds\":[\"RConn1\"],\"side\":\"BOTTOM\"},\"type\":\"ConnectorPlacement.EquallySpacedRectSide\",\"uuid\":\"c37fa533-1c55-4ba2-8511-ae6957d58015\"}]},\"type\":\"ConnectorPlacement.EquallySpacedConnector\",\"uuid\":\"da1ef182-4ed3-4fb4-823f-e8eb0a5ecd15\"}],\"packageUris\":[\"http://schema.mathworks.com/mf0/Connector/R2020b\"],\"version\":\"1.0\"}"
  39X (CABLE) : Subsystem
      settings: PortSchema="{\"entries\":[{\"content\":{\"headerSize\":26,\"margin\":15,\"minimumSpacing\":25,\"sides\":[{\"content\":{},\"type\":\"ConnectorPlacement.EquallySpacedRectSide\",\"uuid\":\"c62bca68-e99b-4d4a-8c3b-c9a3c6520291\"},{\"content\":{\"side\":\"RIGHT\"},\"type\":\"ConnectorPlacement.EquallySpacedRectSide\",\"uuid\":\"9f78cd75-5645-4950-8d66-9f0d33627f1f\"},{\"content\":{\"side\":\"TOP\"},\"type\":\"ConnectorPlacement.EquallySpacedRectSide\",\"uuid\":\"f95077c9-4a6b-4bf1-8b13-59697d659817\"},{\"content\":{\"connectorIds\":[\"RConn1\"],\"side\":\"BOTTOM\"},\"type\":\"ConnectorPlacement.EquallySpacedRectSide\",\"uuid\":\"e78b483f-198f-4f0e-9598-a8b9a7d84052\"}]},\"type\":\"ConnectorPlacement.EquallySpacedConnector\",\"uuid\":\"da1ef182-4ed3-4fb4-823f-e8eb0a5ecd15\"}],\"packageUris\":[\"http://schema.mathworks.com/mf0/Connector/R2020b\"],\"version\":\"1.0\"}"
  14X-30X : PMIOPort  Side=Left
  14X-31X : PMIOPort  Port=2  Side=Left
  14X-32X : PMIOPort  Port=3  Side=Left
  14X-33X : PMIOPort  Port=4  Side=Left
  14X-34X : PMIOPort  Port=5  Side=Left
  14X-35X : PMIOPort  Port=6  Side=Left
  14X-36X : PMIOPort  Port=7  Side=Left
  14X-37X : PMIOPort  Port=8  Side=Left
  14X-38X : PMIOPort  Port=9  Side=Left
  14X-39X : PMIOPort  Port=10  Side=Left
  connections:
  14X-30X/RConn1 -- 30X (LVGS)/RConn1
  14X-31X/RConn1 -- 31X (HVGS)/RConn1
  14X-32X/RConn1 -- 32X (EMER. GS)/RConn1
  14X-33X/RConn1 -- 33X (LVSB)/RConn1
  14X-34X/RConn1 -- 34X (HVSB)/RConn1
  14X-35X/RConn1 -- 35X (TRANSFORMERS)/RConn1
  14X-36X/RConn1 -- 36X (SHORE POWER)/RConn1
  14X-37X/RConn1 -- 37X (BATTERY)/RConn1
  14X-38X/RConn1 -- 38X (FEEDER PANELS)/RConn1
  14X-39X/RConn1 -- 39X (CABLE)/RConn1

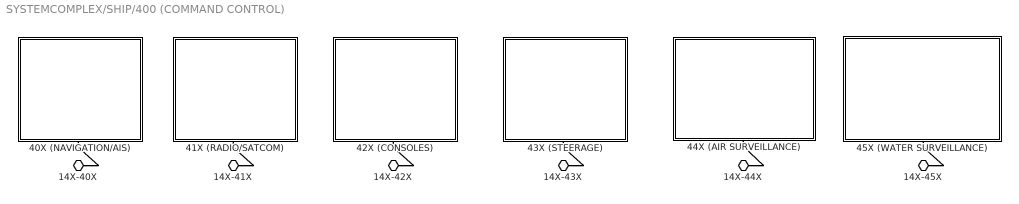
== system SYSTEMCOMPLEX/SHIP/400 (COMMAND CONTROL) ==
  40X (NAVIGATION/AIS) : Subsystem
      settings: PortSchema="{\"entries\":[{\"content\":{\"headerSize\":26,\"margin\":15,\"minimumSpacing\":25,\"sides\":[{\"content\":{},\"type\":\"ConnectorPlacement.EquallySpacedRectSide\",\"uuid\":\"c62bca68-e99b-4d4a-8c3b-c9a3c6520291\"},{\"content\":{\"side\":\"RIGHT\"},\"type\":\"ConnectorPlacement.EquallySpacedRectSide\",\"uuid\":\"9f78cd75-5645-4950-8d66-9f0d33627f1f\"},{\"content\":{\"side\":\"TOP\"},\"type\":\"ConnectorPlacement.EquallySpacedRectSide\",\"uuid\":\"f95077c9-4a6b-4bf1-8b13-59697d659817\"},{\"content\":{\"connectorIds\":[\"RConn1\"],\"side\":\"BOTTOM\"},\"type\":\"ConnectorPlacement.EquallySpacedRectSide\",\"uuid\":\"e935d9f9-aea2-413e-8cf6-9bc030435579\"}]},\"type\":\"ConnectorPlacement.EquallySpacedConnector\",\"uuid\":\"da1ef182-4ed3-4fb4-823f-e8eb0a5ecd15\"}],\"packageUris\":[\"http://schema.mathworks.com/mf0/Connector/R2020b\"],\"version\":\"1.0\"}"
  41X (RADIO/SATCOM) : Subsystem
      settings: PortSchema="{\"entries\":[{\"content\":{\"headerSize\":26,\"margin\":15,\"minimumSpacing\":25,\"sides\":[{\"content\":{},\"type\":\"ConnectorPlacement.EquallySpacedRectSide\",\"uuid\":\"c62bca68-e99b-4d4a-8c3b-c9a3c6520291\"},{\"content\":{\"side\":\"RIGHT\"},\"type\":\"ConnectorPlacement.EquallySpacedRectSide\",\"uuid\":\"9f78cd75-5645-4950-8d66-9f0d33627f1f\"},{\"content\":{\"side\":\"TOP\"},\"type\":\"ConnectorPlacement.EquallySpacedRectSide\",\"uuid\":\"f95077c9-4a6b-4bf1-8b13-59697d659817\"},{\"content\":{\"connectorIds\":[\"RConn1\"],\"side\":\"BOTTOM\"},\"type\":\"ConnectorPlacement.EquallySpacedRectSide\",\"uuid\":\"5cbd5441-aa77-48c3-bdfa-e246717f4108\"}]},\"type\":\"ConnectorPlacement.EquallySpacedConnector\",\"uuid\":\"da1ef182-4ed3-4fb4-823f-e8eb0a5ecd15\"}],\"packageUris\":[\"http://schema.mathworks.com/mf0/Connector/R2020b\"],\"version\":\"1.0\"}"
  42X (CONSOLES) : Subsystem
      settings: PortSchema="{\"entries\":[{\"content\":{\"headerSize\":26,\"margin\":15,\"minimumSpacing\":25,\"sides\":[{\"content\":{},\"type\":\"ConnectorPlacement.EquallySpacedRectSide\",\"uuid\":\"c62bca68-e99b-4d4a-8c3b-c9a3c6520291\"},{\"content\":{\"side\":\"RIGHT\"},\"type\":\"ConnectorPlacement.EquallySpacedRectSide\",\"uuid\":\"9f78cd75-5645-4950-8d66-9f0d33627f1f\"},{\"content\":{\"side\":\"TOP\"},\"type\":\"ConnectorPlacement.EquallySpacedRectSide\",\"uuid\":\"f95077c9-4a6b-4bf1-8b13-59697d659817\"},{\"content\":{\"connectorIds\":[\"RConn1\"],\"side\":\"BOTTOM\"},\"type\":\"ConnectorPlacement.EquallySpacedRectSide\",\"uuid\":\"c5de9276-d9c2-46cf-8c7e-b3f9fb328951\"}]},\"type\":\"ConnectorPlacement.EquallySpacedConnector\",\"uuid\":\"da1ef182-4ed3-4fb4-823f-e8eb0a5ecd15\"}],\"packageUris\":[\"http://schema.mathworks.com/mf0/Connector/R2020b\"],\"version\":\"1.0\"}"
  43X (STEERAGE) : Subsystem
      settings: PortSchema="{\"entries\":[{\"content\":{\"headerSize\":26,\"margin\":15,\"minimumSpacing\":25,\"sides\":[{\"content\":{},\"type\":\"ConnectorPlacement.EquallySpacedRectSide\",\"uuid\":\"c62bca68-e99b-4d4a-8c3b-c9a3c6520291\"},{\"content\":{\"side\":\"RIGHT\"},\"type\":\"ConnectorPlacement.EquallySpacedRectSide\",\"uuid\":\"9f78cd75-5645-4950-8d66-9f0d33627f1f\"},{\"content\":{\"side\":\"TOP\"},\"type\":\"ConnectorPlacement.EquallySpacedRectSide\",\"uuid\":\"f95077c9-4a6b-4bf1-8b13-59697d659817\"},{\"content\":{\"connectorIds\":[\"RConn1\"],\"side\":\"BOTTOM\"},\"type\":\"ConnectorPlacement.EquallySpacedRectSide\",\"uuid\":\"1465ccd5-1a98-48b0-9cd8-36fa76ab4133\"}]},\"type\":\"ConnectorPlacement.EquallySpacedConnector\",\"uuid\":\"da1ef182-4ed3-4fb4-823f-e8eb0a5ecd15\"}],\"packageUris\":[\"http://schema.mathworks.com/mf0/Connector/R2020b\"],\"version\":\"1.0\"}"
  44X (AIR SURVEILLANCE) : Subsystem
      settings: PortSchema="{\"entries\":[{\"content\":{\"headerSize\":26,\"margin\":15,\"minimumSpacing\":25,\"sides\":[{\"content\":{},\"type\":\"ConnectorPlacement.EquallySpacedRectSide\",\"uuid\":\"c62bca68-e99b-4d4a-8c3b-c9a3c6520291\"},{\"content\":{\"side\":\"RIGHT\"},\"type\":\"ConnectorPlacement.EquallySpacedRectSide\",\"uuid\":\"9f78cd75-5645-4950-8d66-9f0d33627f1f\"},{\"content\":{\"side\":\"TOP\"},\"type\":\"ConnectorPlacement.EquallySpacedRectSide\",\"uuid\":\"f95077c9-4a6b-4bf1-8b13-59697d659817\"},{\"content\":{\"connectorIds\":[\"RConn1\"],\"side\":\"BOTTOM\"},\"type\":\"ConnectorPlacement.EquallySpacedRectSide\",\"uuid\":\"6beca900-1c5b-4fac-a3d4-fa1fc7089e4a\"}]},\"type\":\"ConnectorPlacement.EquallySpacedConnector\",\"uuid\":\"da1ef182-4ed3-4fb4-823f-e8eb0a5ecd15\"}],\"packageUris\":[\"http://schema.mathworks.com/mf0/Connector/R2020b\"],\"version\":\"1.0\"}"
  45X (WATER SURVEILLANCE) : Subsystem
      settings: PortSchema="{\"entries\":[{\"content\":{\"headerSize\":26,\"margin\":15,\"minimumSpacing\":25,\"sides\":[{\"content\":{},\"type\":\"ConnectorPlacement.EquallySpacedRectSide\",\"uuid\":\"c62bca68-e99b-4d4a-8c3b-c9a3c6520291\"},{\"content\":{\"side\":\"RIGHT\"},\"type\":\"ConnectorPlacement.EquallySpacedRectSide\",\"uuid\":\"9f78cd75-5645-4950-8d66-9f0d33627f1f\"},{\"content\":{\"side\":\"TOP\"},\"type\":\"ConnectorPlacement.EquallySpacedRectSide\",\"uuid\":\"f95077c9-4a6b-4bf1-8b13-59697d659817\"},{\"content\":{\"connectorIds\":[\"RConn1\"],\"side\":\"BOTTOM\"},\"type\":\"ConnectorPlacement.EquallySpacedRectSide\",\"uuid\":\"7ae0f6cc-ced0-4af9-bc1e-7d0c2c53387e\"}]},\"type\":\"ConnectorPlacement.EquallySpacedConnector\",\"uuid\":\"da1ef182-4ed3-4fb4-823f-e8eb0a5ecd15\"}],\"packageUris\":[\"http://schema.mathworks.com/mf0/Connector/R2020b\"],\"version\":\"1.0\"}"
  14X-40X : PMIOPort  Side=Left
  14X-41X : PMIOPort  Port=2  Side=Left
  14X-42X : PMIOPort  Port=3  Side=Left
  14X-43X : PMIOPort  Port=4  Side=Left
  14X-44X : PMIOPort  Port=5  Side=Left
  14X-45X : PMIOPort  Port=6  Side=Left
  connections:
  14X-40X/RConn1 -- 40X (NAVIGATION/AIS)/RConn1
  14X-41X/RConn1 -- 41X (RADIO/SATCOM)/RConn1
  14X-42X/RConn1 -- 42X (CONSOLES)/RConn1
  14X-43X/RConn1 -- 43X (STEERAGE)/RConn1
  14X-44X/RConn1 -- 44X (AIR SURVEILLANCE)/RConn1
  14X-45X/RConn1 -- 45X (WATER SURVEILLANCE)/RConn1
